simulink model "S_model"  (R2018b)
settings: Solver=VariableStepAuto  StartTime=0.0  StopTime=10.0  RelTol=1e-3
model workspace (MAT data in the model file):
  K = 0.00794
  N1 = 0.00747
  N2 = 0.0958
  alpha = 0.0482
  beta = 0.931
  lambda = 0.0958
settings Model: Creator=rache  LastModifiedBy=rache

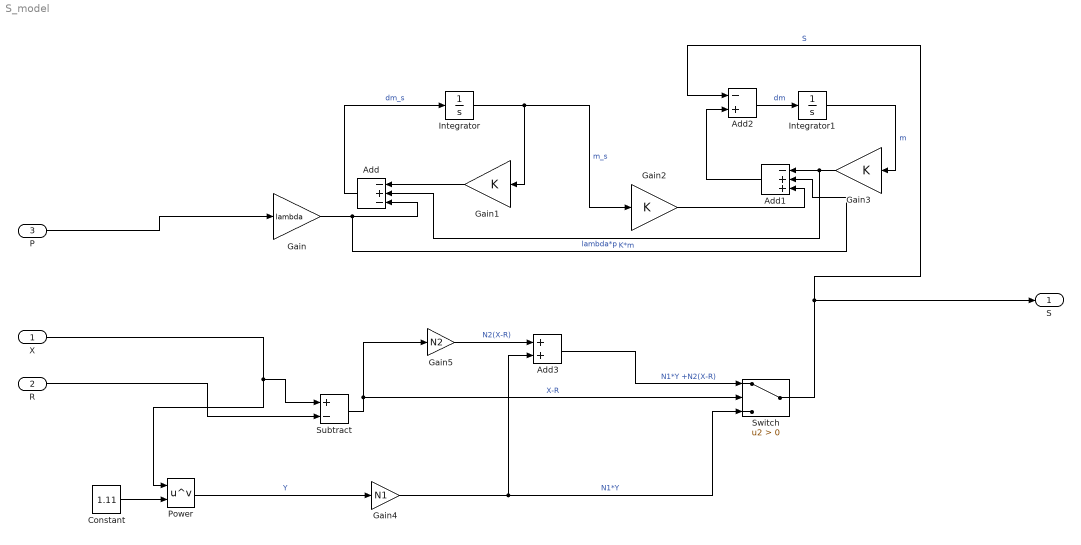
== system S_model ==
  X : Inport
  R : Inport  Port=2
  P : Inport  Port=3
  Add : Sum  Inputs=-+-
  Add1 : Sum  Inputs=-++
  Add2 : Sum  Inputs=-+
  Add3 : Sum
  Constant : Constant  Value=1.11
  Gain : Gain  Gain=lambda
  Gain1 : Gain  Gain=K
  Gain2 : Gain  Gain=K
  Gain3 : Gain  Gain=K
  Gain4 : Gain  Gain=N1
  Gain5 : Gain  Gain=N2
  Integrator : Integrator
  Integrator1 : Integrator
  Power : Math  Operator=pow  SaturateOnIntegerOverflow=on
  Subtract : Sum  Inputs=+-
  Switch : Switch  Criteria=u2 > Threshold
  S : Outport
  wires:
  R/1 -> Subtract/2
  Subtract/1 -> Gain5/1, Switch/2  "X-R"
  P/1 -> Gain/1
  Integrator/1 -> Gain1/1, Gain2/1  "m_s"
  Add/1 -> Integrator/1  "dm_s"
  Gain1/1 -> Add/1
  Gain3/1 -> Add/2, Add1/1  "K*m"
  Integrator1/1 -> Gain3/1  "m"
  Gain/1 -> Add1/2, Add/3  "lambda*p"
  Gain2/1 -> Add1/3
  Add2/1 -> Integrator1/1  "dm"
  Add1/1 -> Add2/2
  Switch/1 -> Add2/1, S/1  "S"
  Constant/1 -> Power/2
  X/1 -> Power/1, Subtract/1
  Power/1 -> Gain4/1  "Y"
  Gain4/1 -> Add3/2, Switch/3  "N1*Y"
  Gain5/1 -> Add3/1  "N2(X-R)"
  Add3/1 -> Switch/1  "N1*Y +N2(X-R)"
